simulink model "wikel_mesung_block"  (R2012b)
settings: Solver=ode45  StartTime=0.0  StopTime=10.0  RelTol=1e-3
libraries: powerlib_extras x2
settings Model: Creator=Nikolay  LastModifiedBy=Nikolay

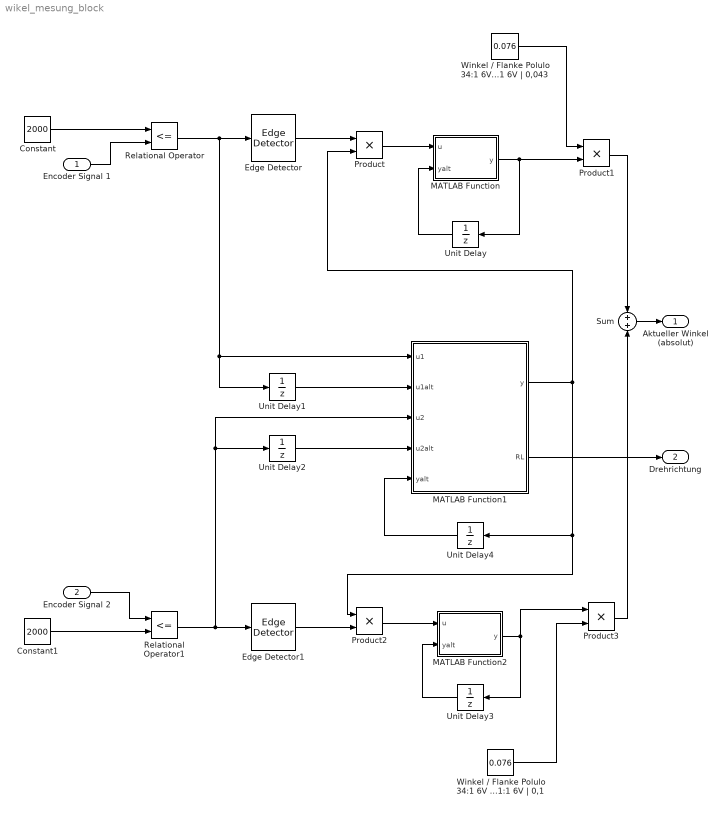
== system wikel_mesung_block ==
  Encoder Signal 1 : Inport
  Encoder Signal 2 : Inport  Port=2
  Constant : Constant  Value=2000
  Constant1 : Constant  Value=2000
  Edge Detector : powerlib_extras/Control  Blocks/Edge Detector  model=Either  ic=0
  Edge Detector1 : powerlib_extras/Control  Blocks/Edge Detector  model=Either  ic=0
  MATLAB Function : MATLAB Function  TreatAsAtomicUnit=on
  MATLAB Function1 : MATLAB Function  TreatAsAtomicUnit=on
  MATLAB Function2 : MATLAB Function  TreatAsAtomicUnit=on
  Product{,1..3} (4 alike) : Product  RndMeth=Zero
  Relational Operator : RelationalOperator  Operator=<=  OutDataTypeStr=boolean
  Relational Operator1 : RelationalOperator  Operator=<=  OutDataTypeStr=boolean
  Sum : Sum
  Unit Delay{,1..4} (5 alike) : UnitDelay  SampleTime=-1
  Winkel / Flanke Polulo 34:1 6V | 0,22 Polulo 74:1 6V | 0,1 Polulo 98:1 6V | 0,076 Polulo 171:1 6V | 0,043 : Constant  Value=0.076
  Winkel / Flanke Polulo 34:1 6V | 0,22 Polulo 74:1 6V | 0,1 Polulo 98:1 6V | 0,076 Polulo 171:1 6V | 0,1 : Constant  Value=0.076
  Aktueller Winkel (absolut) : Outport
  Drehrichtung : Outport  Port=2
  wires:
  Encoder Signal 1/1 -> Relational Operator/2
  Relational Operator/1 -> Edge Detector/1, Unit Delay1/1, MATLAB Function1/1(u1)
  Product/1 -> MATLAB Function/1(u)
  MATLAB Function/1(y) -> Product1/2, Unit Delay/1
  Unit Delay/1 -> MATLAB Function/2(yalt)
  Winkel / Flanke Polulo 34:1 6V | 0,22 Polulo 74:1 6V | 0,1 Polulo 98:1 6V | 0,076 Polulo 171:1 6V | 0,043/1 -> Product1/1
  Product1/1 -> Sum/1
  Sum/1 -> Aktueller Winkel (absolut)/1
  Edge Detector/1 -> Product/1
  Unit Delay1/1 -> MATLAB Function1/2(u1alt)
  Unit Delay2/1 -> MATLAB Function1/4(u2alt)
  Relational Operator1/1 -> Unit Delay2/1, MATLAB Function1/3(u2), Edge Detector1/1
  Product2/1 -> MATLAB Function2/1(u)
  MATLAB Function2/1(y) -> Product3/1, Unit Delay3/1
  Unit Delay3/1 -> MATLAB Function2/2(yalt)
  Winkel / Flanke Polulo 34:1 6V | 0,22 Polulo 74:1 6V | 0,1 Polulo 98:1 6V | 0,076 Polulo 171:1 6V | 0,1/1 -> Product3/2
  Edge Detector1/1 -> Product2/2
  Constant1/1 -> Relational Operator1/2
  Encoder Signal 2/1 -> Relational Operator1/1
  Product3/1 -> Sum/2
  MATLAB Function1/1(y) -> Product2/1, Unit Delay4/1, Product/2
  Unit Delay4/1 -> MATLAB Function1/5(yalt)
  MATLAB Function1/2(RL) -> Drehrichtung/1
  Constant/1 -> Relational Operator/1

== matlab function wikel_mesung_block/MATLAB Function1 ==
  data: u1 input; u1alt input; u2 input; u2alt input; y output; yalt input; RL output
function [y, RL] = fcn(u1, u1alt, u2, u2alt, yalt)

y = 1;
RL = 1;

if u1alt == 0 && u2alt == 0 && u1 == 0 && u2 == 0
    y = yalt;
end

if u1alt == 0 && u2alt == 0 && u1 == 0 && u2 == 1
    y = 1;
end

if u1alt == 0 && u2alt == 0 && u1 == 1 && u2 == 0
    y = -1;
end

% if u1alt == 0 && u2alt == 0 && u1 == 1 && u2 == 1
%     y = yalt;   % nicht mglich
% end

if u1alt == 0 && u2alt == 1 && u1 == 0 && u2 == 0
    y = -1;
end

if u1alt == 0 && u2alt == 1 && u1 == 0 && u2 == 1
    y = yalt;
end

% if u1alt == 0 && u2alt == 1 && u1 == 1 && u2 == 0
%     y = yalt;   % nicht mglich
% end

if u1alt == 0 && u2alt == 1 && u1 == 1 && u2 == 1
    y = 1;
end

if u1alt == 1 && u2alt == 0 && u1 == 0 && u2 == 0
    y = 1;
end

% if u1alt == 1 && u2alt == 0 && u1 == 0 && u2 == 1
%     y = yalt;   % nicht mglich
% end

if u1alt == 1 && u2alt == 0 && u1 == 1 && u2 == 0
    y = yalt;
end

if u1alt == 1 && u2alt == 0 && u1 == 1 && u2 == 1
    y = -1;
end

% if u1alt == 1 && u2alt == 1 && u1 == 0 && u2 == 0
%     y = yalt;   % nicht mglich
% end

if u1alt == 1 && u2alt == 1 && u1 == 0 && u2 == 1
    y = -1;
end

if u1alt == 1 && u2alt == 1 && u1 == 1 && u2 == 0
    y = 1;
end

if u1alt == 1 && u2alt == 1 && u1 == 1 && u2 == 1
    y = yalt;
end

if y == 1
    RL = 1;
else
    RL = 0;
end

== matlab function wikel_mesung_block/MATLAB Function ==
  data: u input; y output; yalt input
function y = fcn(u, yalt)

y = yalt + u;

== matlab function wikel_mesung_block/MATLAB Function2 ==
  data: u input; y output; yalt input
function y = fcn(u, yalt)

y = yalt + u;
